simulink model "AC_Assg_1_Q2"  (R2025b)
settings: Solver=VariableStepAuto  StartTime=0.0  StopTime=10.0  RelTol=1e-3
settings Model: Creator=hale  LastModifiedBy=hale

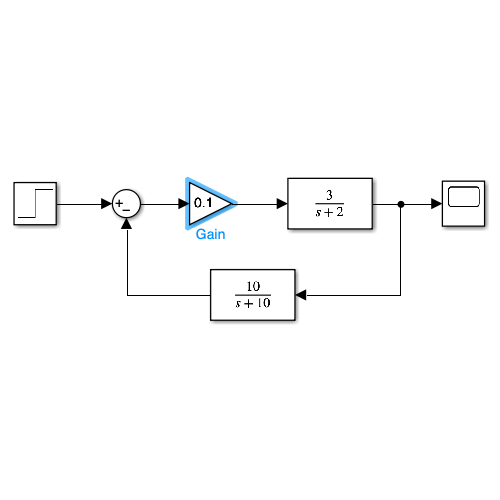
[thumbnail: Simulink's stored preview of the top-level diagram]
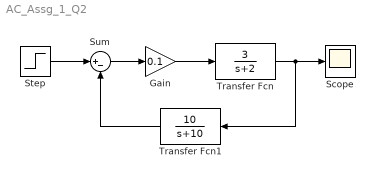
== system AC_Assg_1_Q2 ==
  Gain : Gain  Gain=0.1
  Scope : Scope
      settings: ActiveDisplayYMinimum=-0.016304347818858866  ActiveDisplayYMaximum=0.14673913036972983
  Step : Step  SampleTime=0
  Sum : Sum  Inputs=|+-
  Transfer Fcn : TransferFcn  Numerator=[3]  Denominator=[1 2]
  Transfer Fcn1 : TransferFcn  Numerator=10  Denominator=[1 10]
  wires:
  Step/1 -> Sum/1
  Transfer Fcn/1 -> Transfer Fcn1/1, Scope/1
  Sum/1 -> Gain/1
  Gain/1 -> Transfer Fcn/1
  Transfer Fcn1/1 -> Sum/2
